simulink model "open"  (R2025a)
settings: Solver=VariableStepAuto  StartTime=0.0  StopTime=0.05  MaxStep=1e-9  RelTol=1e-3
libraries: spsVoltageMeasurementLib x5, spsSeriesRLCBranchLib x4, spsCurrentMeasurementLib x4, spsDiodeLib x2, spsMosfetLib x2, spsDCVoltageSourceLib x1, spsLinearTransformerLib x1, sps_lib x1
settings Model: Creator=FCH  LastModifiedBy=FCH
settings DataIOCC: ReturnWorkspaceOutputs=off

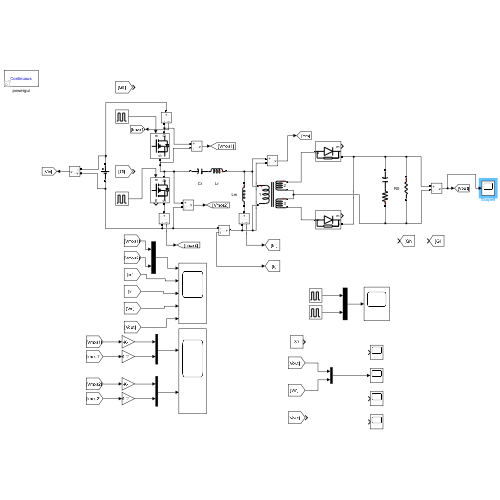
[thumbnail: Simulink's stored preview of the top-level diagram]
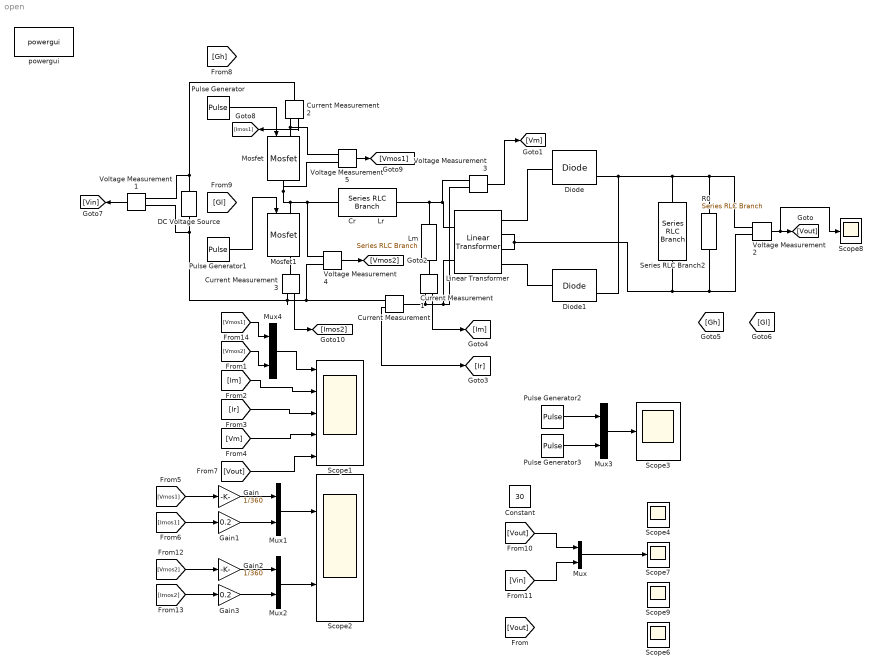
== system open ==
  Constant : Constant  Value=30
  Cr           Lr : spsSeriesRLCBranchLib/Series RLC Branch  LConnTagsString=__new0  RConnTagsString=__new0  BranchType=LC  Resistance=1  Inductance=18e-6  SetiL0=off  InitialCurrent=0  Capacitance=36e-9  Setx0=off  InitialVoltage=0  Measurements=None
  Current Measurement{,1..3} (4 alike) : spsCurrentMeasurementLib/Current Measurement  PhasorSimulation=off  OutputType=Complex  PSBequivalent=0
  DC Voltage Source : spsDCVoltageSourceLib/DC Voltage Source  Amplitude=400  Measurements=None
  Diode : spsDiodeLib/Diode  Ron=0.001  Lon=0  Vf=0.7  IC=0  UseSnubber=0  Rs=500  Cs=250e-9  Measurements=on
  Diode1 : spsDiodeLib/Diode  Ron=0.001  Lon=0  Vf=0.7  IC=0  UseSnubber=0  Rs=500  Cs=250e-9  Measurements=on
  Gain : Gain  Gain=1/360
  Gain1 : Gain  Gain=0.2
  Gain2 : Gain  Gain=1/360
  Gain3 : Gain  Gain=0.2
  Linear Transformer : spsLinearTransformerLib/Linear Transformer  UNITS=SI  NominalPower=[ 250e2 180e3 ]  winding1=[10 0 0]  winding2=[1 0 0]  ThreeWindings=on  winding3=[1 0 0]  RmLm=[inf inf]  Measurements=None  DataType=on
  Lm : spsSeriesRLCBranchLib/Series RLC Branch  LConnTagsString=__new0  RConnTagsString=__new0  BranchType=L  Resistance=1  Inductance=100e-6  SetiL0=off  InitialCurrent=0  Capacitance=1e-6  Setx0=off  InitialVoltage=0  Measurements=None
  Mosfet : spsMosfetLib/Mosfet  Ron=0.1  Lon=0  Rd=0.01  Vfd=0  IC=0  Rs=1e5  Cs=389e-9  Measurements=off
  Mosfet1 : spsMosfetLib/Mosfet  Ron=0.1  Lon=0  Rd=0.01  Vfd=0  IC=0  Rs=1e5  Cs=389e-9  Measurements=on
  Mux{,1..4} (5 alike) : Mux  Inputs=2
  Pulse Generator : DiscretePulseGenerator  PulseType=Time based  Period=1/197.7e3  PulseWidth=50
  Pulse Generator1 : DiscretePulseGenerator  PulseType=Time based  Period=1/197.7e3  PulseWidth=50  PhaseDelay=180/360*1/197.7e3
  Pulse Generator2 : DiscretePulseGenerator  PulseType=Time based  Period=1/270e3  PulseWidth=45
  Pulse Generator3 : DiscretePulseGenerator  PulseType=Time based  Period=1/270e3  PulseWidth=45  PhaseDelay=180/360*1/270e3
  R0 : spsSeriesRLCBranchLib/Series RLC Branch  LConnTagsString=__new0  RConnTagsString=__new0  BranchType=R  Resistance=10000  Inductance=1e-3  SetiL0=off  InitialCurrent=0  Capacitance=1e-6  Setx0=off  InitialVoltage=0  Measurements=Branch voltage
  Scope1 : Scope  NumInputPorts=5
      settings: ActiveDisplayYMinimum=-50.027810234382422  ActiveDisplayYMaximum=450.02781023438246
  Scope2 : Scope  NumInputPorts=2
      settings: ActiveDisplayYMinimum=-0.61361587322765931  ActiveDisplayYMaximum=1.3876265656966265
  Scope{3..4,6..9} (6 alike) : Scope
      Scope3 settings: ActiveDisplayYMinimum=-0.26664494974207453  ActiveDisplayYMaximum=1.2272147750858355  DataLoggingVariableName=ScopeData3
      Scope4 settings: ActiveDisplayYMinimum=199635.39769332195  ActiveDisplayYMaximum=227972.22664518646  DataLoggingVariableName=ScopeData4
      Scope6 settings: ActiveDisplayYMinimum=-44.999999999999972  ActiveDisplayYMaximum=404.99999999999994  DataLoggingVariableName=ScopeData6
      Scope7 settings: ActiveDisplayYMinimum=-44.999999999999972  ActiveDisplayYMaximum=404.99999999999994  DataLoggingVariableName=ScopeData2
      Scope8 settings: ActiveDisplayYMinimum=23.7464416284072  ActiveDisplayYMaximum=23.766805582403379  DataLoggingVariableName=U_output
      Scope9 settings: ActiveDisplayYMinimum=-25.704316529059234  ActiveDisplayYMaximum=36.189368503228835  DataLoggingVariableName=ScopeData8
  Series RLC Branch2 : spsSeriesRLCBranchLib/Series RLC Branch  LConnTagsString=__new0  RConnTagsString=__new0  BranchType=RC  Resistance=0.01  Inductance=1e-3  SetiL0=off  InitialCurrent=0  Capacitance=1e-6  Setx0=off  InitialVoltage=0  Measurements=None
  Voltage Measurement{1..5} (5 alike) : spsVoltageMeasurementLib/Voltage Measurement  PhasorSimulation=off  OutputType=Complex  PSBequivalent=0
  powergui : sps_lib/powergui  Priority=1  SimulationMode=Continuous  SampleTime=1/(200e6)  frequency=60  Iterations=50  frequencyindice=0  Pbase=100e6  ErrMax=1e-4  UnitsV=kV  UnitsW=MW  buscounter=0  FunctionMessages=off  echomessages=off  EnableUseOfTLC=off  CurrentSourceSwitches=off  DisableSnubberDevices=off  DisableRonSwitches=off  DisableVfSwitches=off  DisplayEquations=off  AutomaticDiscreteSolvers=off  SolverType=Tustin/Backward Euler (TBE)  Interpol=off  ExternalGateDelay=off  methode=off  Ts=100  x0status=blocks  SPID=on  SwTol=0  HookPort=off  NonlinearTolerance=1e-4  nMaxIteration=100  ContinueOnMaxIteration=off  RestoreLinks=warning  ResistiveCurrentMeasurement=off  Frange=[0:2:500]  Ylog=off  Xlog=on  ShowGrid=off  save=off  variable=ZData  structure=0  ZoomFFT=off  StartTime=0.0  cycles=1  DisplayStyle=1  fundamental=60  FreqAxis=off  MaxFrequency=1000  frequencyindicesteady=1  RmsSteady=1  display=off
  wires:
  Voltage Measurement2/1 -> Scope8/1, [Vout]
  Voltage Measurement3/1 -> [Vm]
  Voltage Measurement4/1 -> [Vmos2]
  Current Measurement/1 -> [Ir]
  Current Measurement1/1 -> [Im]
  [Im] -> Scope1/2
  [Ir] -> Scope1/3
  [Vm] -> Scope1/4
  [Vout] -> Scope1/5
  Mux/1 -> Scope7/1
  [Vout] -> Mux/1
  Voltage Measurement1/1 -> [Vin]
  [Vin] -> Mux/2
  Current Measurement2/1 -> [Imos1]
  Voltage Measurement5/1 -> [Vmos1]
  Current Measurement3/1 -> [Imos2]
  [Vmos1] -> Gain/1
  [Imos1] -> Gain1/1
  Mux1/1 -> Scope2/1
  [Vmos2] -> Gain2/1
  [Imos2] -> Gain3/1
  Mux2/1 -> Scope2/2
  Gain/1 -> Mux1/1
  Gain1/1 -> Mux1/2
  Gain2/1 -> Mux2/1
  Gain3/1 -> Mux2/2
  Pulse Generator/1 -> Mosfet/1
  Pulse Generator1/1 -> Mosfet1/1
  Pulse Generator2/1 -> Mux3/1
  Pulse Generator3/1 -> Mux3/2
  Mux3/1 -> Scope3/1
  [Vmos2] -> Mux4/2
  [Vmos1] -> Mux4/1
  Mux4/1 -> Scope1/1
  connections:
  DC Voltage Source/RConn1 -- Voltage Measurement1/LConn2 -- Current Measurement2/LConn1
  Mosfet/RConn1 -- Voltage Measurement4/LConn1 -- Cr           Lr/RConn1 -- Mosfet1/LConn1 -- Voltage Measurement5/LConn2
  Lm/RConn1 -- Current Measurement1/LConn1
  Cr           Lr/LConn1 -- Voltage Measurement3/LConn1 -- Linear Transformer/LConn1 -- Lm/LConn1
  Linear Transformer/RConn1 -- Diode/LConn1
  Diode/RConn1 -- Diode1/RConn1 -- Series RLC Branch2/RConn1 -- R0/LConn1 -- Voltage Measurement2/LConn1
  R0/RConn1 -- Voltage Measurement2/LConn2 -- Linear Transformer/RConn2 -- Linear Transformer/RConn3 -- Series RLC Branch2/LConn1
  Linear Transformer/RConn4 -- Diode1/LConn1
  Current Measurement/RConn1 -- Voltage Measurement1/LConn1 -- DC Voltage Source/LConn1 -- Current Measurement3/RConn1 -- Voltage Measurement4/LConn2
  Linear Transformer/LConn2 -- Voltage Measurement3/LConn2 -- Current Measurement1/RConn1 -- Current Measurement/LConn1
  Current Measurement2/RConn1 -- Mosfet/LConn1 -- Voltage Measurement5/LConn1
  Mosfet1/RConn1 -- Current Measurement3/LConn1
